simulink model "CM640A_MotAg1Meas"  (R2013b)
settings: Solver=FixedStepDiscrete  SolverMode=SingleTasking  StartTime=0.0  StopTime=1  FixedStep=0.0000625  RelTol=1e-3
undefined symbols (not defined in the file): ARCHGLBPRM_2PI_ULS_F32, COEFFTBLELMSIZE_CNT_U08, COEFFTBLSIZE_CNT_U08, CORRNTBLAGSTEPSIZE_MATRAD_F32, CORRNTBLSIDXOFFS_CNT_U16, CORRNTBLSIZE_CNT_U16, CORRNTBLSIZEMASK_CNT_U08, MOTAG1OFFS_MOTREV_U0P16, MotAg1PrtclFlt, MOTAG1PRTCLFLTFAILSTEP_CNT_U16, MOTAG1PRTCLFLTPASSSTEP_CNT_U16, MOTAGDELTAPERCORRNPT_CNT_U16, MOTAGIDXMASK_CNT_U16, MotCtrlMotAg1ErrReg, NtcSts1, sigbuilder_block, SNSRAGMASK_CNT_U32, SNSRERRMASK_CNT_U32, SNSRERRNTCMASK_CNT_U08, SNSRVLTGFLTMASK_CNT_U32, SPIPARMASK_CNT_U32
libraries: simulink x28, FloatToFixd x1, NxtrMax x1, NxtrLim x1
(part 3 of 4)

== system CM640A_MotAg1Meas/MotAg1Meas/MotAg1MeasInit1/Compute Correction Table/NVM Ok/Calculate Correction Table/Build Wave ==
  Constant : Constant  Value=CORRNTBLSIZE_CNT_U16
  CopyRight2 : Subsystem  Description=|  mask(Copyright Information){none=on}
      | Copyright info block.                                               
      |                                                                     
      | Place copyright information at the top of every subsystem in design.
      mask prompts: none "No parameters"
      mask help: Place copyright information at the top of every subsystem in design.
      mask Display:
      | NxtrConf = 'Nexteer Confidential';
      | 
      | sys = bdroot; %handle for the current model ("system")
      | first = get_param(sys,'Created');
      | first = first(end-3:end);  %year is last four digits
      | 
      | last = get_param(sys,'LastModifiedDate');
      | if isempty(last)
      |     last = datestr(now,'yyyy');
      | else
      |     last = last(end-3:end);
      | end
      | 
      | if strcmp(first,last)
      |     fprintf('%s -- Copyright %s Nexteer',NxtrConf,first)
      | else
      |     fprintf('%s -- %s%s- %s Nexteer',NxtrConf,char(169),first,last)
      | end
  Reconstructed Waveform Processing : Subsystem  TreatAsAtomicUnit=on
  wires:
  Constant/1 -> Reconstructed Waveform Processing/1(N)

== system CM640A_MotAg1Meas/MotAg1Meas/MotAg1MeasInit1/Compute Correction Table/NVM Ok/Calculate Correction Table/Change Correction Coordinate ==
  Constant1 : Constant  Value=CORRNTBLSIZE_CNT_U16
  CopyRight2 : Subsystem  Description=|  mask(Copyright Information){none=on}
      | Copyright info block.                                               
      |                                                                     
      | Place copyright information at the top of every subsystem in design.
      mask prompts: none "No parameters"
      mask help: Place copyright information at the top of every subsystem in design.
      mask Display:
      | NxtrConf = 'Nexteer Confidential';
      | 
      | sys = bdroot; %handle for the current model ("system")
      | first = get_param(sys,'Created');
      | first = first(end-3:end);  %year is last four digits
      | 
      | last = get_param(sys,'LastModifiedDate');
      | if isempty(last)
      |     last = datestr(now,'yyyy');
      | else
      |     last = last(end-3:end);
      | end
      | 
      | if strcmp(first,last)
      |     fprintf('%s -- Copyright %s Nexteer',NxtrConf,first)
      | else
      |     fprintf('%s -- %s%s- %s Nexteer',NxtrConf,char(169),first,last)
      | end
  Waveform Coordinate Change : Subsystem  TreatAsAtomicUnit=on
  wires:
  Constant1/1 -> Waveform Coordinate Change/1(N)

== system CM640A_MotAg1Meas/MotAg1Meas/MotAg1MeasInit1/Compute Correction Table/NVM Ok/Calculate Correction Table/CopyRight2 ==

== system CM640A_MotAg1Meas/MotAg1Meas/MotAg1MeasInit1/Compute Correction Table/NVM Ok/Configure Coefficients/CopyRight2 ==

== system CM640A_MotAg1Meas/MotAg1Meas/MotAg1MeasPer1/Process MotAg1 Angle/Process MotAg1Raw/MotAg Message Parity Monitoring/Atomic Subsystem2 ==
  InputBoolean : Inport  OutDataTypeStr=boolean
  If : If  IfExpression=u1 ~= 0
  Merge : Merge
  Output 0 : Subsystem  TreatAsAtomicUnit=on
  Output 1 : Subsystem  TreatAsAtomicUnit=on
  OutputNumber : Outport  OutDataTypeStr=uint8
  wires:
  InputBoolean/1 -> If/1
  If/1 -> Output 1/Action
  If/2 -> Output 0/Action
  Output 1/1(Out1) -> Merge/1
  Output 0/1(Out1) -> Merge/2
  Merge/1 -> OutputNumber/1

== system CM640A_MotAg1Meas/MotAg1Meas/MotAg1MeasPer1/Process MotAg1 Angle/Process MotAg1Raw/MotAg Message Parity Monitoring/Atomic Subsystem3 ==
  InputBoolean : Inport  OutDataTypeStr=boolean
  If : If  IfExpression=u1 ~= 0
  Merge : Merge
  Output 0 : Subsystem  TreatAsAtomicUnit=on
  Output 1 : Subsystem  TreatAsAtomicUnit=on
  OutputNumber : Outport  OutDataTypeStr=uint8
  wires:
  Merge/1 -> OutputNumber/1
  Output 0/1(Out1) -> Merge/2
  Output 1/1(Out1) -> Merge/1
  If/2 -> Output 0/Action
  If/1 -> Output 1/Action
  InputBoolean/1 -> If/1

== system CM640A_MotAg1Meas/MotAg1Meas/MotAg1MeasPer1/Process MotAg1 Angle/Process MotAg1Raw/MotAg Message Parity Monitoring/CopyRight2 ==

== system CM640A_MotAg1Meas/MotAg1Meas/MotAg1MeasPer1/Process MotAg1 Angle/Process MotAg1Raw/Raw Mecl Mot Ag Processing/CopyRight2 ==

== system CM640A_MotAg1Meas/MotAg1Meas/MotAg1MeasPer1/Process MotAg1 Angle/Process MotAg1Raw/Undervoltage Bit Monitoring/Atomic Subsystem1 ==
  InputBoolean : Inport  OutDataTypeStr=boolean
  If : If  IfExpression=u1 ~= 0
  Merge : Merge
  Output 0 : Subsystem  TreatAsAtomicUnit=on
  Output 1 : Subsystem  TreatAsAtomicUnit=on
  OutputNumber : Outport  OutDataTypeStr=uint8
  wires:
  InputBoolean/1 -> If/1
  If/1 -> Output 1/Action
  If/2 -> Output 0/Action
  Output 1/1(Out1) -> Merge/1
  Output 0/1(Out1) -> Merge/2
  Merge/1 -> OutputNumber/1

== system CM640A_MotAg1Meas/MotAg1Meas/MotAg1MeasPer1/Process MotAg1 Angle/Process MotAg1Raw/Undervoltage Bit Monitoring/CopyRight2 ==

== system CM640A_MotAg1Meas/MotAg1Meas/MotAg1MeasPer2/MotAg1 Protocol Fault Operation/Atomic Subsystem/N Step/CopyRight2 ==

== system CM640A_MotAg1Meas/MotAg1Meas/MotAg1MeasPer2/MotAg1 Protocol Fault Operation/Atomic Subsystem/P Step/CopyRight2 ==

== system CM640A_MotAg1Meas/MotAg1Meas/MotAg1MeasPer2/MotAg1 Protocol Fault Operation/Subsystem/Atomic Subsystem1/Output 0 ==
  Action Port : ActionPort  ActionType=else
  Bit 7 : Constant  Value=0  OutDataTypeStr=uint8
  Out1 : Outport  InitialOutput=0
  wires:
  Bit 7/1 -> Out1/1

== system CM640A_MotAg1Meas/MotAg1Meas/MotAg1MeasPer2/MotAg1 Protocol Fault Operation/Subsystem/Atomic Subsystem1/Output 1 ==
  Action Port : ActionPort  ActionType=then
  Bit 7 : Constant  OutDataTypeStr=uint8
  Out1 : Outport  InitialOutput=1
  wires:
  Bit 7/1 -> Out1/1

== system CM640A_MotAg1Meas/MotAg1Meas/MotAg1MeasPer2/MotAg1 Protocol Fault Operation/Subsystem/Atomic Subsystem2/Output 0 ==
  Action Port : ActionPort  ActionType=else
  Bit 7 : Constant  Value=0  OutDataTypeStr=uint8
  Out1 : Outport  InitialOutput=0
  wires:
  Bit 7/1 -> Out1/1

== system CM640A_MotAg1Meas/MotAg1Meas/MotAg1MeasPer2/MotAg1 Protocol Fault Operation/Subsystem/Atomic Subsystem2/Output 1 ==
  Action Port : ActionPort  ActionType=then
  Bit 7 : Constant  OutDataTypeStr=uint8
  Out1 : Outport  InitialOutput=1
  wires:
  Bit 7/1 -> Out1/1

== system CM640A_MotAg1Meas/MotAg1Meas/MotAg1MeasPer2/MotAg1 Protocol Fault Operation/Subsystem/Atomic Subsystem3/Output 0 ==
  Action Port : ActionPort  ActionType=else
  Bit 7 : Constant  Value=0  OutDataTypeStr=uint8
  Out1 : Outport  InitialOutput=0
  wires:
  Bit 7/1 -> Out1/1

== system CM640A_MotAg1Meas/MotAg1Meas/MotAg1MeasPer2/MotAg1 Protocol Fault Operation/Subsystem/Atomic Subsystem3/Output 1 ==
  Action Port : ActionPort  ActionType=then
  Bit 7 : Constant  OutDataTypeStr=uint8
  Out1 : Outport  InitialOutput=1
  wires:
  Bit 7/1 -> Out1/1

== system CM640A_MotAg1Meas/MotAg1Meas/MotAg1MeasPer2/Process ErrorReg and DieRevCtr/Process MotAg1RawErr/Invalid Polarity, Hold Last Value/CopyRight2 ==

== system CM640A_MotAg1Meas/MotAg1Meas/MotAg1MeasPer2/Process ErrorReg and DieRevCtr/Process MotAg1RawErr/Process MotAg1RawErr/Atomic Subsystem1 ==
  InputBoolean : Inport  OutDataTypeStr=boolean
  If : If  IfExpression=u1 ~= 0
  Merge : Merge
  Output 0 : Subsystem  TreatAsAtomicUnit=on
  Output 1 : Subsystem  TreatAsAtomicUnit=on
  OutputNumber : Outport  OutDataTypeStr=uint8
  wires:
  InputBoolean/1 -> If/1
  If/1 -> Output 1/Action
  If/2 -> Output 0/Action
  Output 1/1(Out1) -> Merge/1
  Output 0/1(Out1) -> Merge/2
  Merge/1 -> OutputNumber/1

== system CM640A_MotAg1Meas/MotAg1Meas/MotAg1MeasPer2/Process ErrorReg and DieRevCtr/Process MotAg1RawErr/Process MotAg1RawErr/Atomic Subsystem2 ==
  InputBoolean : Inport  OutDataTypeStr=boolean
  If : If  IfExpression=u1 ~= 0
  Merge : Merge
  Output 0 : Subsystem  TreatAsAtomicUnit=on
  Output 1 : Subsystem  TreatAsAtomicUnit=on
  OutputNumber : Outport  OutDataTypeStr=uint8
  wires:
  Merge/1 -> OutputNumber/1
  Output 0/1(Out1) -> Merge/2
  Output 1/1(Out1) -> Merge/1
  If/2 -> Output 0/Action
  If/1 -> Output 1/Action
  InputBoolean/1 -> If/1

== system CM640A_MotAg1Meas/MotAg1Meas/MotAg1MeasPer2/Process ErrorReg and DieRevCtr/Process MotAg1RawErr/Process MotAg1RawErr/CopyRight2 ==

== system CM640A_MotAg1Meas/MotAg1Meas/MotAg1MeasPer2/Process ErrorReg and DieRevCtr/Process MotAg1RawErr/Valid Polarity/CopyRight2 ==

== system CM640A_MotAg1Meas/MotAg1Meas/MotAg1MeasInit1/Compute Correction Table/NVM Ok/Calculate Correction Table/Build Wave/CopyRight2 ==

== system CM640A_MotAg1Meas/MotAg1Meas/MotAg1MeasInit1/Compute Correction Table/NVM Ok/Calculate Correction Table/Build Wave/Reconstructed Waveform Processing ==
  N : Inport
  Assignment : Assignment  IndexMode=Zero-based  IndexOptions=Index vector (port)  Indices=1  OutputSizes=1
  Constant : Constant  Value=COEFFTBLSIZE_CNT_U08
  Constant1 : Constant  Value=CORRNTBLAGSTEPSIZE_MATRAD_F32
  CopyRight2 : Subsystem  Description=|  mask(Copyright Information){none=on}
      | Copyright info block.                                               
      |                                                                     
      | Place copyright information at the top of every subsystem in design.
      mask prompts: none "No parameters"
      mask help: Place copyright information at the top of every subsystem in design.
      mask Display:
      | NxtrConf = 'Nexteer Confidential';
      | 
      | sys = bdroot; %handle for the current model ("system")
      | first = get_param(sys,'Created');
      | first = first(end-3:end);  %year is last four digits
      | 
      | last = get_param(sys,'LastModifiedDate');
      | if isempty(last)
      |     last = datestr(now,'yyyy');
      | else
      |     last = last(end-3:end);
      | end
      | 
      | if strcmp(first,last)
      |     fprintf('%s -- Copyright %s Nexteer',NxtrConf,first)
      | else
      |     fprintf('%s -- %s%s- %s Nexteer',NxtrConf,char(169),first,last)
      | end
  Data Store Read : DataStoreRead  DataStoreName=ReconstructedWaveform_RevM_f32
  Data Store Write : DataStoreWrite  DataStoreName=ReconstructedWaveform_RevM_f32
  Data Type Conversion : DataTypeConversion  OutDataTypeStr=single
  Data Type Conversion1 : DataTypeConversion  OutDataTypeStr=int8
  For Iterator : ForIterator  ResetStates=reset  IterationSource=external  IndexMode=Zero-based  IterationVariableDataType=int16
  Harmonic Coefficient Processing : Subsystem  TreatAsAtomicUnit=on
  Product : Product
  Subtract 1 because the first order is not included : Bias  Bias=-1
  wires:
  Constant/1 -> Data Type Conversion1/1
  N/1 -> For Iterator/1
  For Iterator/1 -> Data Type Conversion/1, Assignment/3
  Data Type Conversion/1 -> Product/1
  Constant1/1 -> Product/2
  Product/1 -> Harmonic Coefficient Processing/1(HarmAngle)
  Subtract 1 because the first order is not included/1 -> Harmonic Coefficient Processing/2(Coefficient Table Size)
  Data Type Conversion1/1 -> Subtract 1 because the first order is not included/1
  Harmonic Coefficient Processing/1(Reconstructed Waveform Element) -> Assignment/2
  Data Store Read/1 -> Assignment/1
  Assignment/1 -> Data Store Write/1

== system CM640A_MotAg1Meas/MotAg1Meas/MotAg1MeasInit1/Compute Correction Table/NVM Ok/Calculate Correction Table/Change Correction Coordinate/CopyRight2 ==

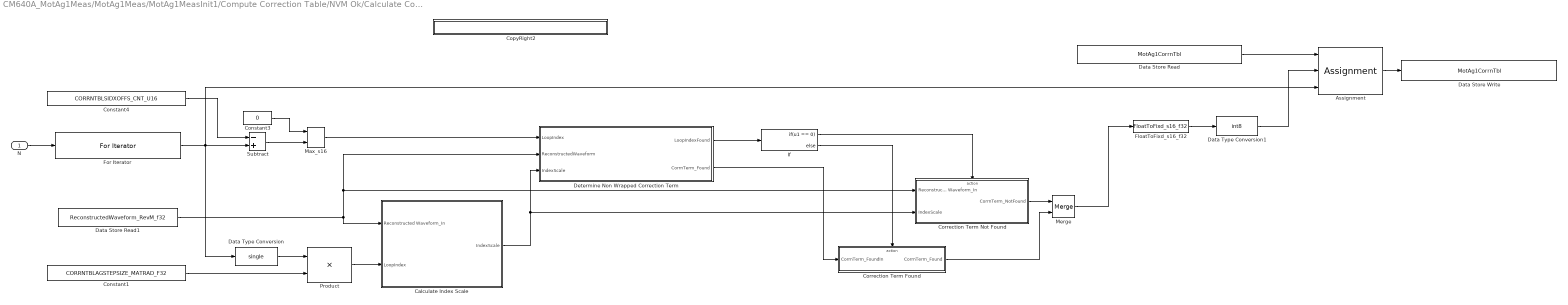
== system CM640A_MotAg1Meas/MotAg1Meas/MotAg1MeasInit1/Compute Correction Table/NVM Ok/Calculate Correction Table/Change Correction Coordinate/Waveform Coordinate Change ==
  N : Inport
  Assignment : Assignment  IndexMode=Zero-based  IndexOptions=Index vector (port)  Indices=1  OutputSizes=1
  Calculate Index Scale : Subsystem  TreatAsAtomicUnit=on
  Constant1 : Constant  Value=CORRNTBLAGSTEPSIZE_MATRAD_F32
  Constant3 : Constant  Value=0  OutDataTypeStr=int16
  Constant4 : Constant  Value=CORRNTBLSIDXOFFS_CNT_U16
  CopyRight2 : Subsystem  Description=|  mask(Copyright Information){none=on}
      | Copyright info block.                                               
      |                                                                     
      | Place copyright information at the top of every subsystem in design.
      mask prompts: none "No parameters"
      mask help: Place copyright information at the top of every subsystem in design.
      mask Display:
      | NxtrConf = 'Nexteer Confidential';
      | 
      | sys = bdroot; %handle for the current model ("system")
      | first = get_param(sys,'Created');
      | first = first(end-3:end);  %year is last four digits
      | 
      | last = get_param(sys,'LastModifiedDate');
      | if isempty(last)
      |     last = datestr(now,'yyyy');
      | else
      |     last = last(end-3:end);
      | end
      | 
      | if strcmp(first,last)
      |     fprintf('%s -- Copyright %s Nexteer',NxtrConf,first)
      | else
      |     fprintf('%s -- %s%s- %s Nexteer',NxtrConf,char(169),first,last)
      | end
  Correction Term Found : Subsystem  TreatAsAtomicUnit=on
  Correction Term Not Found : Subsystem  TreatAsAtomicUnit=on
  Data Store Read : DataStoreRead  DataStoreName=MotAg1CorrnTbl
  Data Store Read1 : DataStoreRead  DataStoreName=ReconstructedWaveform_RevM_f32
  Data Store Write : DataStoreWrite  DataStoreName=MotAg1CorrnTbl
  Data Type Conversion : DataTypeConversion  OutDataTypeStr=single
  Data Type Conversion1 : DataTypeConversion  OutDataTypeStr=int8
  Determine Non Wrapped Correction Term : Subsystem  TreatAsAtomicUnit=on
  FloatToFixd_s16_f32 : FloatToFixd/FloatToFixd_s16_f32  Param1=12
  For Iterator : ForIterator  ResetStates=reset  IterationSource=external  IndexMode=Zero-based  IterationVariableDataType=int16
  If : If  IfExpression=u1 == 0
  Max_s16 : NxtrMax/Max_s16  SFunctionSpec="int16 y1 = Max_s16( int16 u1,  int16 u2)"
      settings: AttributesFormatString=%<Name>
  Merge : Merge
  Product : Product
  Subtract : Sum  Inputs=-+  OutDataTypeStr=int16
  wires:
  Constant1/1 -> Product/2
  Data Type Conversion/1 -> Product/1
  For Iterator/1 -> Data Type Conversion/1, Assignment/3, Subtract/2
  N/1 -> For Iterator/1
  Data Store Read1/1 -> Calculate Index Scale/1(Reconstructed Waveform_In), Correction Term Not Found/1(Reconstructed Waveform_In), Determine Non Wrapped Correction Term/2(ReconstructedWaveform)
  Product/1 -> Calculate Index Scale/2(LoopIndex)
  Calculate Index Scale/1(IndexScale) -> Correction Term Not Found/2(IndexScale), Determine Non Wrapped Correction Term/3(IndexScale)
  Constant3/1 -> Max_s16/1
  Subtract/1 -> Max_s16/2
  Constant4/1 -> Subtract/1
  Max_s16/1 -> Determine Non Wrapped Correction Term/1(LoopIndex)
  Determine Non Wrapped Correction Term/1(LoopIndexFound) -> If/1
  If/1 -> Correction Term Not Found/Action
  If/2 -> Correction Term Found/Action
  Determine Non Wrapped Correction Term/2(CorrnTerm_Found) -> Correction Term Found/1(CorrnTerm_FoundIn)
  Data Store Read/1 -> Assignment/1
  Correction Term Not Found/1(CorrnTerm_NotFound) -> Merge/1
  Correction Term Found/1(CorrnTerm_Found) -> Merge/2
  Merge/1 -> FloatToFixd_s16_f32/1
  Assignment/1 -> Data Store Write/1
  FloatToFixd_s16_f32/1 -> Data Type Conversion1/1
  Data Type Conversion1/1 -> Assignment/2

== system CM640A_MotAg1Meas/MotAg1Meas/MotAg1MeasPer1/Process MotAg1 Angle/Process MotAg1Raw/MotAg Message Parity Monitoring/Atomic Subsystem2/Output 0 ==
  Action Port : ActionPort  ActionType=else
  Bit 7 : Constant  Value=0  OutDataTypeStr=uint8
  Out1 : Outport  InitialOutput=0
  wires:
  Bit 7/1 -> Out1/1

== system CM640A_MotAg1Meas/MotAg1Meas/MotAg1MeasPer1/Process MotAg1 Angle/Process MotAg1Raw/MotAg Message Parity Monitoring/Atomic Subsystem2/Output 1 ==
  Action Port : ActionPort  ActionType=then
  Bit 7 : Constant  OutDataTypeStr=uint8
  Out1 : Outport  InitialOutput=1
  wires:
  Bit 7/1 -> Out1/1

== system CM640A_MotAg1Meas/MotAg1Meas/MotAg1MeasPer1/Process MotAg1 Angle/Process MotAg1Raw/MotAg Message Parity Monitoring/Atomic Subsystem3/Output 0 ==
  Action Port : ActionPort  ActionType=else
  Bit 7 : Constant  Value=0  OutDataTypeStr=uint8
  Out1 : Outport  InitialOutput=0
  wires:
  Bit 7/1 -> Out1/1

== system CM640A_MotAg1Meas/MotAg1Meas/MotAg1MeasPer1/Process MotAg1 Angle/Process MotAg1Raw/MotAg Message Parity Monitoring/Atomic Subsystem3/Output 1 ==
  Action Port : ActionPort  ActionType=then
  Bit 7 : Constant  OutDataTypeStr=uint8
  Out1 : Outport  InitialOutput=1
  wires:
  Bit 7/1 -> Out1/1

== system CM640A_MotAg1Meas/MotAg1Meas/MotAg1MeasPer1/Process MotAg1 Angle/Process MotAg1Raw/Undervoltage Bit Monitoring/Atomic Subsystem1/Output 0 ==
  Action Port : ActionPort  ActionType=else
  Bit 7 : Constant  Value=0  OutDataTypeStr=uint8
  Out1 : Outport  InitialOutput=0
  wires:
  Bit 7/1 -> Out1/1

== system CM640A_MotAg1Meas/MotAg1Meas/MotAg1MeasPer1/Process MotAg1 Angle/Process MotAg1Raw/Undervoltage Bit Monitoring/Atomic Subsystem1/Output 1 ==
  Action Port : ActionPort  ActionType=then
  Bit 7 : Constant  OutDataTypeStr=uint8
  Out1 : Outport  InitialOutput=1
  wires:
  Bit 7/1 -> Out1/1

== system CM640A_MotAg1Meas/MotAg1Meas/MotAg1MeasPer2/Process ErrorReg and DieRevCtr/Process MotAg1RawErr/Process MotAg1RawErr/Atomic Subsystem1/Output 0 ==
  Action Port : ActionPort  ActionType=else
  Bit 7 : Constant  Value=0  OutDataTypeStr=uint8
  Out1 : Outport  InitialOutput=0
  wires:
  Bit 7/1 -> Out1/1

== system CM640A_MotAg1Meas/MotAg1Meas/MotAg1MeasPer2/Process ErrorReg and DieRevCtr/Process MotAg1RawErr/Process MotAg1RawErr/Atomic Subsystem1/Output 1 ==
  Action Port : ActionPort  ActionType=then
  Bit 7 : Constant  OutDataTypeStr=uint8
  Out1 : Outport  InitialOutput=1
  wires:
  Bit 7/1 -> Out1/1

== system CM640A_MotAg1Meas/MotAg1Meas/MotAg1MeasPer2/Process ErrorReg and DieRevCtr/Process MotAg1RawErr/Process MotAg1RawErr/Atomic Subsystem2/Output 0 ==
  Action Port : ActionPort  ActionType=else
  Bit 7 : Constant  Value=0  OutDataTypeStr=uint8
  Out1 : Outport  InitialOutput=0
  wires:
  Bit 7/1 -> Out1/1

== system CM640A_MotAg1Meas/MotAg1Meas/MotAg1MeasPer2/Process ErrorReg and DieRevCtr/Process MotAg1RawErr/Process MotAg1RawErr/Atomic Subsystem2/Output 1 ==
  Action Port : ActionPort  ActionType=then
  Bit 7 : Constant  OutDataTypeStr=uint8
  Out1 : Outport  InitialOutput=1
  wires:
  Bit 7/1 -> Out1/1

== system CM640A_MotAg1Meas/MotAg1Meas/MotAg1MeasInit1/Compute Correction Table/NVM Ok/Calculate Correction Table/Build Wave/Reconstructed Waveform Processing/CopyRight2 ==

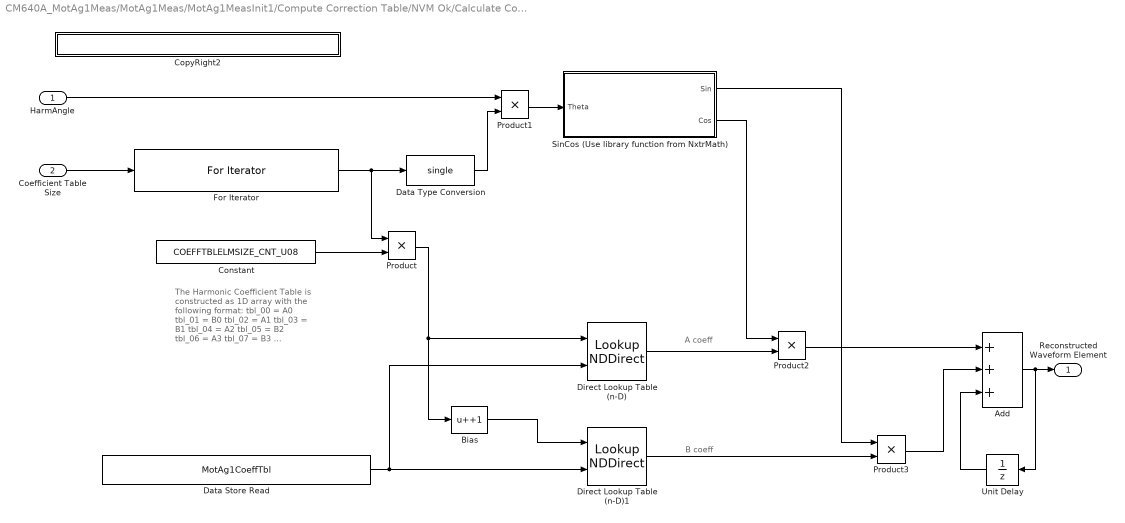
== system CM640A_MotAg1Meas/MotAg1Meas/MotAg1MeasInit1/Compute Correction Table/NVM Ok/Calculate Correction Table/Build Wave/Reconstructed Waveform Processing/Harmonic Coefficient Processing ==
  note: B coeff
  note: A coeff
  note: The Harmonic Coefficient Table
      | is constructed as 1D array with
      | the following format:
      |
      | tbl_00 = A0
      | tbl_01 = B0
      | tbl_02 = A1
      | tbl_03 = B1
      | tbl_04 = A2
      | tbl_05 = B2
      | tbl_06 = A3
      | tbl_07 = B3
      | ...
  HarmAngle : Inport
  Coefficient Table Size : Inport  Port=2
  Add : Sum  Inputs=+++
  Bias : Bias  Bias=+1
  Constant : Constant  Value=COEFFTBLELMSIZE_CNT_U08
  CopyRight2 : Subsystem  Description=|  mask(Copyright Information){none=on}
      | Copyright info block.                                               
      |                                                                     
      | Place copyright information at the top of every subsystem in design.
      mask prompts: none "No parameters"
      mask help: Place copyright information at the top of every subsystem in design.
      mask Display:
      | NxtrConf = 'Nexteer Confidential';
      | 
      | sys = bdroot; %handle for the current model ("system")
      | first = get_param(sys,'Created');
      | first = first(end-3:end);  %year is last four digits
      | 
      | last = get_param(sys,'LastModifiedDate');
      | if isempty(last)
      |     last = datestr(now,'yyyy');
      | else
      |     last = last(end-3:end);
      | end
      | 
      | if strcmp(first,last)
      |     fprintf('%s -- Copyright %s Nexteer',NxtrConf,first)
      | else
      |     fprintf('%s -- %s%s- %s Nexteer',NxtrConf,char(169),first,last)
      | end
  Data Store Read : DataStoreRead  DataStoreName=MotAg1CoeffTbl
  Data Type Conversion : DataTypeConversion  OutDataTypeStr=single
  Direct Lookup Table (n-D) : LookupNDDirect  NumberOfTableDimensions=1  TableIsInput=on
  Direct Lookup Table (n-D)1 : LookupNDDirect  NumberOfTableDimensions=1  TableIsInput=on
  For Iterator : ForIterator  ResetStates=reset  IterationSource=external  IterationVariableDataType=int8
  Product{,1..3} (4 alike) : Product
  SinCos (Use library function from NxtrMath) : Subsystem  TreatAsAtomicUnit=on
  Unit Delay : UnitDelay  SampleTime=-1
  Reconstructed Waveform Element : Outport
  wires:
  Coefficient Table Size/1 -> For Iterator/1
  Data Store Read/1 -> Direct Lookup Table (n-D)/2, Direct Lookup Table (n-D)1/2
  Constant/1 -> Product/2
  For Iterator/1 -> Data Type Conversion/1, Product/1
  HarmAngle/1 -> Product1/1
  Data Type Conversion/1 -> Product1/2
  Product1/1 -> SinCos (Use library function from NxtrMath)/1(Theta)
  Product/1 -> Bias/1, Direct Lookup Table (n-D)/1
  Bias/1 -> Direct Lookup Table (n-D)1/1
  SinCos (Use library function from NxtrMath)/2(Cos) -> Product2/1
  Direct Lookup Table (n-D)/1 -> Product2/2
  Direct Lookup Table (n-D)1/1 -> Product3/2
  SinCos (Use library function from NxtrMath)/1(Sin) -> Product3/1
  Product2/1 -> Add/1
  Product3/1 -> Add/2
  Unit Delay/1 -> Add/3
  Add/1 -> Unit Delay/1, Reconstructed Waveform Element/1

== system CM640A_MotAg1Meas/MotAg1Meas/MotAg1MeasInit1/Compute Correction Table/NVM Ok/Calculate Correction Table/Change Correction Coordinate/Waveform Coordinate Change/Calculate Index Scale ==
  Reconstructed Waveform_In : Inport
  LoopIndex : Inport  Port=2
  CopyRight2 : Subsystem  Description=|  mask(Copyright Information){none=on}
      | Copyright info block.                                               
      |                                                                     
      | Place copyright information at the top of every subsystem in design.
      mask prompts: none "No parameters"
      mask help: Place copyright information at the top of every subsystem in design.
      mask Display:
      | NxtrConf = 'Nexteer Confidential';
      | 
      | sys = bdroot; %handle for the current model ("system")
      | first = get_param(sys,'Created');
      | first = first(end-3:end);  %year is last four digits
      | 
      | last = get_param(sys,'LastModifiedDate');
      | if isempty(last)
      |     last = datestr(now,'yyyy');
      | else
      |     last = last(end-3:end);
      | end
      | 
      | if strcmp(first,last)
      |     fprintf('%s -- Copyright %s Nexteer',NxtrConf,first)
      | else
      |     fprintf('%s -- %s%s- %s Nexteer',NxtrConf,char(169),first,last)
      | end
  Direct Lookup Table (n-D) : LookupNDDirect  NumberOfTableDimensions=1  TableIsInput=on
  First Entry Index : Constant  Value=0
  First Entry Index1 : Constant  Value=ARCHGLBPRM_2PI_ULS_F32
  Truth Table : Truth Table  TreatAsAtomicUnit=on
  IndexScale : Outport
  wires:
  Reconstructed Waveform_In/1 -> Direct Lookup Table (n-D)/2
  First Entry Index/1 -> Direct Lookup Table (n-D)/1
  Direct Lookup Table (n-D)/1 -> Truth Table/1(ReconWfrm_0)
  LoopIndex/1 -> Truth Table/2(LoopIndex)
  First Entry Index1/1 -> Truth Table/3(ARCHGLBPRM_2PI_ULS_F32)
  Truth Table/1(IndexScale) -> IndexScale/1

== system CM640A_MotAg1Meas/MotAg1Meas/MotAg1MeasInit1/Compute Correction Table/NVM Ok/Calculate Correction Table/Change Correction Coordinate/Waveform Coordinate Change/CopyRight2 ==

== system CM640A_MotAg1Meas/MotAg1Meas/MotAg1MeasInit1/Compute Correction Table/NVM Ok/Calculate Correction Table/Change Correction Coordinate/Waveform Coordinate Change/Correction Term Found ==
  CorrnTerm_FoundIn : Inport
  Action Port : ActionPort  ActionType=else
  CopyRight2 : Subsystem  Description=|  mask(Copyright Information){none=on}
      | Copyright info block.                                               
      |                                                                     
      | Place copyright information at the top of every subsystem in design.
      mask prompts: none "No parameters"
      mask help: Place copyright information at the top of every subsystem in design.
      mask Display:
      | NxtrConf = 'Nexteer Confidential';
      | 
      | sys = bdroot; %handle for the current model ("system")
      | first = get_param(sys,'Created');
      | first = first(end-3:end);  %year is last four digits
      | 
      | last = get_param(sys,'LastModifiedDate');
      | if isempty(last)
      |     last = datestr(now,'yyyy');
      | else
      |     last = last(end-3:end);
      | end
      | 
      | if strcmp(first,last)
      |     fprintf('%s -- Copyright %s Nexteer',NxtrConf,first)
      | else
      |     fprintf('%s -- %s%s- %s Nexteer',NxtrConf,char(169),first,last)
      | end
  CorrnTerm_Found : Outport
  wires:
  CorrnTerm_FoundIn/1 -> CorrnTerm_Found/1

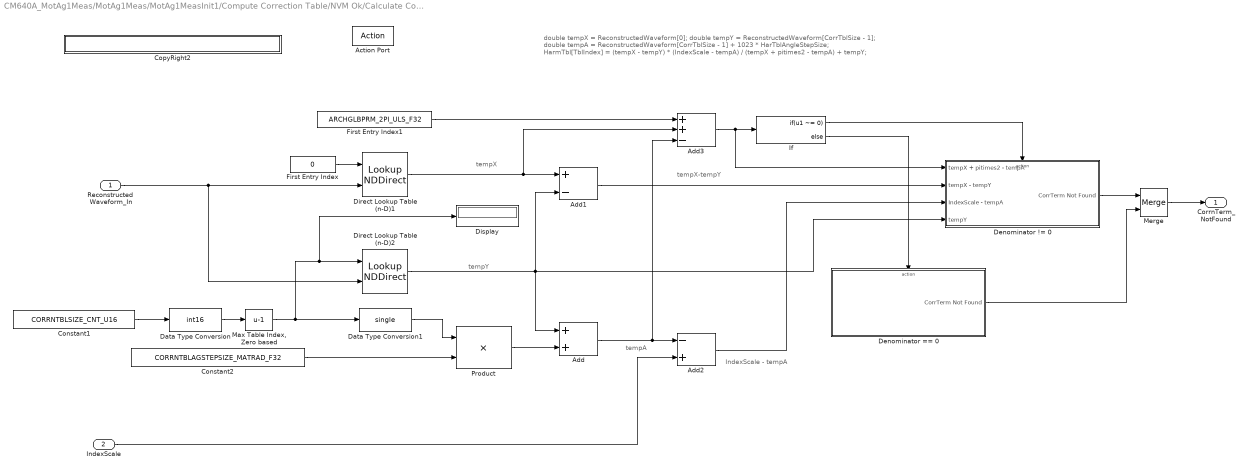
== system CM640A_MotAg1Meas/MotAg1Meas/MotAg1MeasInit1/Compute Correction Table/NVM Ok/Calculate Correction Table/Change Correction Coordinate/Waveform Coordinate Change/Correction Term Not Found ==
  note: double tempX = ReconstructedWaveform[0];
      | double tempY = ReconstructedWaveform[CorrTblSize - 1];
      | double tempA = ReconstructedWaveform[CorrTblSize - 1] + 1023 * HarTblAngleStepSize;
      |
      | HarmTbl[TblIndex] = (tempX - tempY) * (IndexScale - tempA) / (tempX + pitimes2 - tempA) + tempY;
  note: tempX-tempY
  note: IndexScale - tempA
  note: tempA
  note: tempX
  note: tempY
  Reconstructed Waveform_In : Inport  OutDataTypeStr=single
  IndexScale : Inport  Port=2
  Action Port : ActionPort  ActionType=then
  Add : Sum
  Add1 : Sum  Inputs=+-
  Add2 : Sum  Inputs=-+
  Add3 : Sum  Inputs=++-
  Constant1 : Constant  Value=CORRNTBLSIZE_CNT_U16
  Constant2 : Constant  Value=CORRNTBLAGSTEPSIZE_MATRAD_F32
  CopyRight2 : Subsystem  Description=|  mask(Copyright Information){none=on}
      | Copyright info block.                                               
      |                                                                     
      | Place copyright information at the top of every subsystem in design.
      mask prompts: none "No parameters"
      mask help: Place copyright information at the top of every subsystem in design.
      mask Display:
      | NxtrConf = 'Nexteer Confidential';
      | 
      | sys = bdroot; %handle for the current model ("system")
      | first = get_param(sys,'Created');
      | first = first(end-3:end);  %year is last four digits
      | 
      | last = get_param(sys,'LastModifiedDate');
      | if isempty(last)
      |     last = datestr(now,'yyyy');
      | else
      |     last = last(end-3:end);
      | end
      | 
      | if strcmp(first,last)
      |     fprintf('%s -- Copyright %s Nexteer',NxtrConf,first)
      | else
      |     fprintf('%s -- %s%s- %s Nexteer',NxtrConf,char(169),first,last)
      | end
  Data Type Conversion : DataTypeConversion  OutDataTypeStr=int16
  Data Type Conversion1 : DataTypeConversion  OutDataTypeStr=single
  Denominator != 0 : Subsystem  TreatAsAtomicUnit=on
  Denominator == 0 : Subsystem  TreatAsAtomicUnit=on
  Direct Lookup Table (n-D)1 : LookupNDDirect  NumberOfTableDimensions=1  TableIsInput=on
  Direct Lookup Table (n-D)2 : LookupNDDirect  NumberOfTableDimensions=1  TableIsInput=on
  Display : Display
  First Entry Index : Constant  Value=0
  First Entry Index1 : Constant  Value=ARCHGLBPRM_2PI_ULS_F32
  If : If  IfExpression=u1 ~= 0
  "Max Table Index, Zero based" : Bias  Bias=-1
  Merge : Merge
  Product : Product
  CorrnTerm_NotFound : Outport
  wires:
  Reconstructed Waveform_In/1 -> Direct Lookup Table (n-D)2/2, Direct Lookup Table (n-D)1/2
  First Entry Index/1 -> Direct Lookup Table (n-D)1/1
  Constant2/1 -> Product/2
  Constant1/1 -> Data Type Conversion/1
  "Max Table Index, Zero based"/1 -> Data Type Conversion1/1, Display/1, Direct Lookup Table (n-D)2/1
  Data Type Conversion/1 -> "Max Table Index, Zero based"/1
  Data Type Conversion1/1 -> Product/1
  Product/1 -> Add/2
  Direct Lookup Table (n-D)1/1 -> Add3/2, Add1/1
  Add/1 -> Add3/3, Add2/1
  IndexScale/1 -> Add2/2
  First Entry Index1/1 -> Add3/1
  Direct Lookup Table (n-D)2/1 -> Add/1, Denominator != 0/4(tempY), Add1/2
  Add2/1 -> Denominator != 0/3(IndexScale - tempA)
  Add1/1 -> Denominator != 0/2(tempX - tempY)
  Add3/1 -> If/1, Denominator != 0/1(tempX + pitimes2 - tempA)
  If/1 -> Denominator != 0/Action
  If/2 -> Denominator == 0/Action
  Denominator == 0/1(CorrTerm Not Found) -> Merge/2
  Denominator != 0/1(CorrTerm Not Found) -> Merge/1
  Merge/1 -> CorrnTerm_NotFound/1

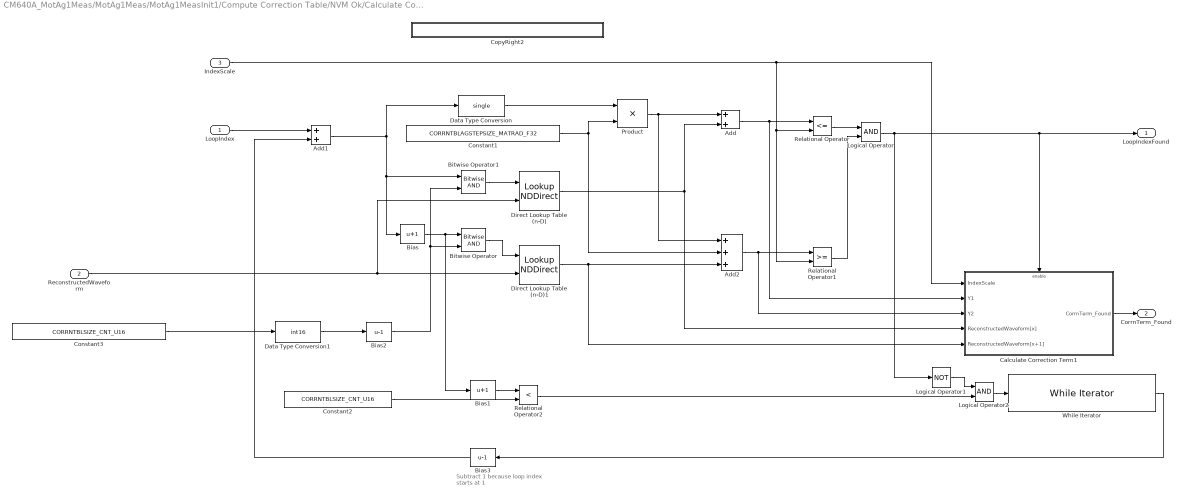
== system CM640A_MotAg1Meas/MotAg1Meas/MotAg1MeasInit1/Compute Correction Table/NVM Ok/Calculate Correction Table/Change Correction Coordinate/Waveform Coordinate Change/Determine Non Wrapped Correction Term ==
  note: Subtract 1 because
      | loop index starts at 1
  LoopIndex : Inport
  ReconstructedWaveform : Inport  Port=2
  IndexScale : Inport  Port=3
  Add : Sum
  Add1 : Sum
  Add2 : Sum  Inputs=+++
  Bias : Bias  Bias=1
  Bias1 : Bias  Bias=1
  Bias2 : Bias  Bias=-1
  Bias3 : Bias  Bias=-1
  Bitwise Operator : simulink/Logic and Bit Operations/Bitwise Operator  logicop=AND  UseBitMask=off  NumInputPorts=2  BitMask=CORRNTBLSIZE_CNT_U16-1  BitMaskRealWorld=Stored Integer
  Bitwise Operator1 : simulink/Logic and Bit Operations/Bitwise Operator  logicop=AND  UseBitMask=off  NumInputPorts=2  BitMask=CORRNTBLSIZE_CNT_U16-1  BitMaskRealWorld=Stored Integer
  Calculate Correction Term1 : Subsystem  TreatAsAtomicUnit=on
  Constant1 : Constant  Value=CORRNTBLAGSTEPSIZE_MATRAD_F32
  Constant2 : Constant  Value=CORRNTBLSIZE_CNT_U16
  Constant3 : Constant  Value=CORRNTBLSIZE_CNT_U16
  CopyRight2 : Subsystem  Description=|  mask(Copyright Information){none=on}
      | Copyright info block.                                               
      |                                                                     
      | Place copyright information at the top of every subsystem in design.
      mask prompts: none "No parameters"
      mask help: Place copyright information at the top of every subsystem in design.
      mask Display:
      | NxtrConf = 'Nexteer Confidential';
      | 
      | sys = bdroot; %handle for the current model ("system")
      | first = get_param(sys,'Created');
      | first = first(end-3:end);  %year is last four digits
      | 
      | last = get_param(sys,'LastModifiedDate');
      | if isempty(last)
      |     last = datestr(now,'yyyy');
      | else
      |     last = last(end-3:end);
      | end
      | 
      | if strcmp(first,last)
      |     fprintf('%s -- Copyright %s Nexteer',NxtrConf,first)
      | else
      |     fprintf('%s -- %s%s- %s Nexteer',NxtrConf,char(169),first,last)
      | end
  Data Type Conversion : DataTypeConversion  OutDataTypeStr=single
  Data Type Conversion1 : DataTypeConversion  OutDataTypeStr=int16
  Direct Lookup Table (n-D) : LookupNDDirect  NumberOfTableDimensions=1  TableIsInput=on
  Direct Lookup Table (n-D)1 : LookupNDDirect  NumberOfTableDimensions=1  TableIsInput=on
  Logical Operator : Logic  AllPortsSameDT=off  OutDataTypeStr=boolean
  Logical Operator1 : Logic  Operator=NOT  AllPortsSameDT=off  OutDataTypeStr=boolean
  Logical Operator2 : Logic  AllPortsSameDT=off  OutDataTypeStr=boolean
  Product : Product
  Relational Operator : RelationalOperator  Operator=<=  OutDataTypeStr=boolean
  Relational Operator1 : RelationalOperator  OutDataTypeStr=boolean
  Relational Operator2 : RelationalOperator  Operator=<  OutDataTypeStr=boolean
  While Iterator : WhileIterator  MaxIters=128  WhileBlockType=do-while  ShowIterationPort=on  OutputDataType=int16
      settings: AttributesFormatString=|
      | Max Iterations:
      | %<MaxIters>
      | (CORRNTBLSIZE_CNT_U16)
  LoopIndexFound : Outport
  CorrnTerm_Found : Outport  Port=2
  wires:
  ReconstructedWaveform/1 -> Direct Lookup Table (n-D)/2, Direct Lookup Table (n-D)1/2
  Add1/1 -> Data Type Conversion/1, Bias/1, Bitwise Operator1/1
  Bias/1 -> Bias1/1, Bitwise Operator/1
  Data Type Conversion/1 -> Product/1
  Product/1 -> Add2/1, Add/1
  Direct Lookup Table (n-D)/1 -> Calculate Correction Term1/4(ReconstructedWaveform[x]), Add/2
  LoopIndex/1 -> Add1/1
  Constant1/1 -> Add2/2, Product/2
  Direct Lookup Table (n-D)1/1 -> Calculate Correction Term1/5(ReconstructedWaveform[x+1]), Add2/3
  Add/1 -> Calculate Correction Term1/2(Y1), Relational Operator/1
  IndexScale/1 -> Calculate Correction Term1/1(IndexScale), Relational Operator1/2, Relational Operator/2
  Add2/1 -> Calculate Correction Term1/3(Y2), Relational Operator1/1
  Relational Operator/1 -> Logical Operator/1
  Relational Operator1/1 -> Logical Operator/2
  Logical Operator/1 -> LoopIndexFound/1, Calculate Correction Term1/Enable, Logical Operator1/1
  Bitwise Operator/1 -> Direct Lookup Table (n-D)1/1
  Bitwise Operator1/1 -> Direct Lookup Table (n-D)/1
  Calculate Correction Term1/1(CorrnTerm_Found) -> CorrnTerm_Found/1
  Logical Operator1/1 -> Logical Operator2/1
  Relational Operator2/1 -> Logical Operator2/2
  Logical Operator2/1 -> While Iterator/1
  Constant2/1 -> Relational Operator2/2
  Bias1/1 -> Relational Operator2/1
  While Iterator/1 -> Bias3/1
  Bias3/1 -> Add1/2
  Constant3/1 -> Data Type Conversion1/1
  Data Type Conversion1/1 -> Bias2/1
  Bias2/1 -> Bitwise Operator1/2, Bitwise Operator/2

== system CM640A_MotAg1Meas/MotAg1Meas/MotAg1MeasInit1/Compute Correction Table/NVM Ok/Calculate Correction Table/Build Wave/Reconstructed Waveform Processing/Harmonic Coefficient Processing/CopyRight2 ==

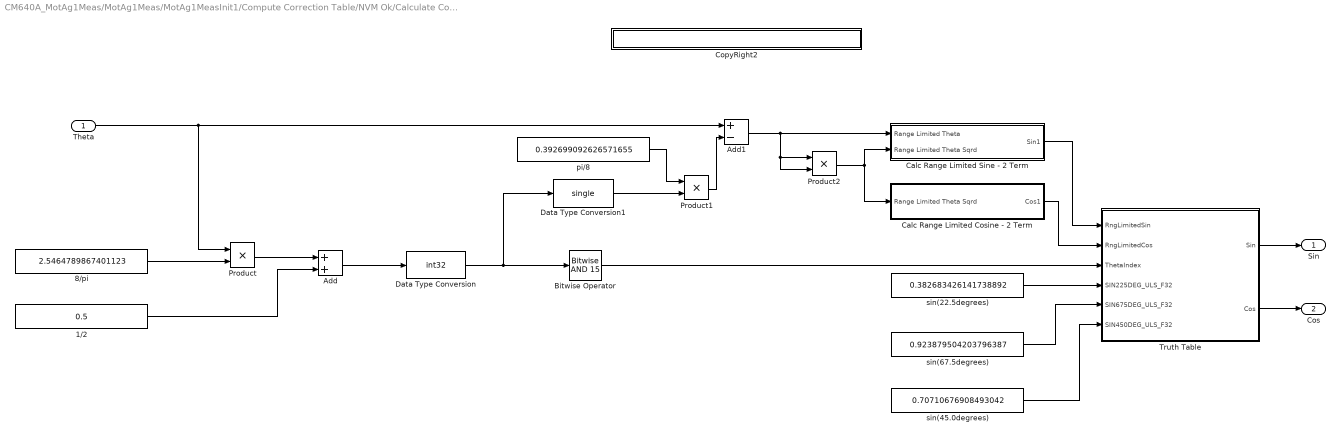
== system CM640A_MotAg1Meas/MotAg1Meas/MotAg1MeasInit1/Compute Correction Table/NVM Ok/Calculate Correction Table/Build Wave/Reconstructed Waveform Processing/Harmonic Coefficient Processing/SinCos (Use library function from NxtrMath) ==
  Theta : Inport
  1/2 : Constant  Value=0.5  OutDataTypeStr=single
  8/pi : Constant  Value=2.5464789867401123  OutDataTypeStr=single
  Add : Sum
  Add1 : Sum  Inputs=+-
  Bitwise Operator : simulink/Logic and Bit Operations/Bitwise Operator  logicop=AND  UseBitMask=on  BitMask=15  BitMaskRealWorld=Stored Integer
      settings: AttributesFormatString=|
      | BitMask:
      | %<BitMask>
  Calc Range Limited Cosine - 2 Term : Subsystem  TreatAsAtomicUnit=on
  Calc Range Limited Sine - 2 Term : Subsystem  TreatAsAtomicUnit=on
  CopyRight2 : Subsystem  Description=|  mask(Copyright Information){none=on}
      | Copyright info block.                                               
      |                                                                     
      | Place copyright information at the top of every subsystem in design.
      mask prompts: none "No parameters"
      mask help: Place copyright information at the top of every subsystem in design.
      mask Display:
      | NxtrConf = 'Nexteer Confidential';
      | 
      | sys = bdroot; %handle for the current model ("system")
      | first = get_param(sys,'Created');
      | first = first(end-3:end);  %year is last four digits
      | 
      | last = get_param(sys,'LastModifiedDate');
      | if isempty(last)
      |     last = datestr(now,'yyyy');
      | else
      |     last = last(end-3:end);
      | end
      | 
      | if strcmp(first,last)
      |     fprintf('%s -- Copyright %s Nexteer',NxtrConf,first)
      | else
      |     fprintf('%s -- %s%s- %s Nexteer',NxtrConf,char(169),first,last)
      | end
  Data Type Conversion : DataTypeConversion  OutDataTypeStr=int32
      settings: AttributesFormatString=Round Method: %<RndMeth>
  Data Type Conversion1 : DataTypeConversion  OutDataTypeStr=single
      settings: AttributesFormatString=Round Method: %<RndMeth>
  Product : Product
  Product1 : Product
  Product2 : Product
  Truth Table : Truth Table  TreatAsAtomicUnit=on
  pi/8 : Constant  Value=0.392699092626571655  OutDataTypeStr=single
  sin(22.5degrees) : Constant  Value=0.382683426141738892  OutDataTypeStr=single
  sin(45.0degrees) : Constant  Value=0.70710676908493042  OutDataTypeStr=single
  sin(67.5degrees) : Constant  Value=0.923879504203796387  OutDataTypeStr=single
  Sin : Outport
  Cos : Outport  Port=2
  wires:
  Theta/1 -> Product/1, Add1/1
  8/pi/1 -> Product/2
  Product/1 -> Add/1
  1/2/1 -> Add/2
  Add/1 -> Data Type Conversion/1
  Data Type Conversion/1 -> Data Type Conversion1/1, Bitwise Operator/1
  pi/8/1 -> Product1/1
  Data Type Conversion1/1 -> Product1/2
  Add1/1 -> Product2/2, Product2/1, Calc Range Limited Sine - 2 Term/1(Range Limited Theta)
  Product1/1 -> Add1/2
  Truth Table/1(Sin) -> Sin/1
  Bitwise Operator/1 -> Truth Table/3(ThetaIndex)
  sin(22.5degrees)/1 -> Truth Table/4(SIN225DEG_ULS_F32)
  sin(67.5degrees)/1 -> Truth Table/5(SIN675DEG_ULS_F32)
  sin(45.0degrees)/1 -> Truth Table/6(SIN450DEG_ULS_F32)
  Product2/1 -> Calc Range Limited Sine - 2 Term/2(Range Limited Theta Sqrd), Calc Range Limited Cosine - 2 Term/1(Range Limited Theta Sqrd)
  Truth Table/2(Cos) -> Cos/1
  Calc Range Limited Sine - 2 Term/1(Sin1) -> Truth Table/1(RngLimitedSin)
  Calc Range Limited Cosine - 2 Term/1(Cos1) -> Truth Table/2(RngLimitedCos)

== system CM640A_MotAg1Meas/MotAg1Meas/MotAg1MeasInit1/Compute Correction Table/NVM Ok/Calculate Correction Table/Change Correction Coordinate/Waveform Coordinate Change/Calculate Index Scale/CopyRight2 ==

== system CM640A_MotAg1Meas/MotAg1Meas/MotAg1MeasInit1/Compute Correction Table/NVM Ok/Calculate Correction Table/Change Correction Coordinate/Waveform Coordinate Change/Correction Term Found/CopyRight2 ==

== system CM640A_MotAg1Meas/MotAg1Meas/MotAg1MeasInit1/Compute Correction Table/NVM Ok/Calculate Correction Table/Change Correction Coordinate/Waveform Coordinate Change/Correction Term Not Found/CopyRight2 ==

== system CM640A_MotAg1Meas/MotAg1Meas/MotAg1MeasInit1/Compute Correction Table/NVM Ok/Calculate Correction Table/Change Correction Coordinate/Waveform Coordinate Change/Correction Term Not Found/Denominator != 0 ==
  note: (tempX - tempY) * (IndexScale - tempA) / (tempX + pitimes2 - tempA)
  note: tempY
  tempX + pitimes2 - tempA : Inport
  tempX - tempY : Inport  Port=2
  IndexScale - tempA : Inport  Port=3
  tempY : Inport  Port=4
  Action Port : ActionPort  ActionType=then
  Add4 : Sum
  CopyRight2 : Subsystem  Description=|  mask(Copyright Information){none=on}
      | Copyright info block.                                               
      |                                                                     
      | Place copyright information at the top of every subsystem in design.
      mask prompts: none "No parameters"
      mask help: Place copyright information at the top of every subsystem in design.
      mask Display:
      | NxtrConf = 'Nexteer Confidential';
      | 
      | sys = bdroot; %handle for the current model ("system")
      | first = get_param(sys,'Created');
      | first = first(end-3:end);  %year is last four digits
      | 
      | last = get_param(sys,'LastModifiedDate');
      | if isempty(last)
      |     last = datestr(now,'yyyy');
      | else
      |     last = last(end-3:end);
      | end
      | 
      | if strcmp(first,last)
      |     fprintf('%s -- Copyright %s Nexteer',NxtrConf,first)
      | else
      |     fprintf('%s -- %s%s- %s Nexteer',NxtrConf,char(169),first,last)
      | end
  "Max Table Index, Zero based1" : Bias
  Product2 : Product  Inputs=/**
  CorrTerm Not Found : Outport
  wires:
  Product2/1 -> Add4/1
  Add4/1 -> "Max Table Index, Zero based1"/1
  "Max Table Index, Zero based1"/1 -> CorrTerm Not Found/1
  tempX + pitimes2 - tempA/1 -> Product2/1
  tempX - tempY/1 -> Product2/2
  IndexScale - tempA/1 -> Product2/3
  tempY/1 -> Add4/2

== system CM640A_MotAg1Meas/MotAg1Meas/MotAg1MeasInit1/Compute Correction Table/NVM Ok/Calculate Correction Table/Change Correction Coordinate/Waveform Coordinate Change/Correction Term Not Found/Denominator == 0 ==
  Action Port : ActionPort  ActionType=else
  Constant : Constant  Value=0  OutDataTypeStr=single
  CopyRight2 : Subsystem  Description=|  mask(Copyright Information){none=on}
      | Copyright info block.                                               
      |                                                                     
      | Place copyright information at the top of every subsystem in design.
      mask prompts: none "No parameters"
      mask help: Place copyright information at the top of every subsystem in design.
      mask Display:
      | NxtrConf = 'Nexteer Confidential';
      | 
      | sys = bdroot; %handle for the current model ("system")
      | first = get_param(sys,'Created');
      | first = first(end-3:end);  %year is last four digits
      | 
      | last = get_param(sys,'LastModifiedDate');
      | if isempty(last)
      |     last = datestr(now,'yyyy');
      | else
      |     last = last(end-3:end);
      | end
      | 
      | if strcmp(first,last)
      |     fprintf('%s -- Copyright %s Nexteer',NxtrConf,first)
      | else
      |     fprintf('%s -- %s%s- %s Nexteer',NxtrConf,char(169),first,last)
      | end
  CorrTerm Not Found : Outport
  wires:
  Constant/1 -> CorrTerm Not Found/1

== system CM640A_MotAg1Meas/MotAg1Meas/MotAg1MeasInit1/Compute Correction Table/NVM Ok/Calculate Correction Table/Change Correction Coordinate/Waveform Coordinate Change/Determine Non Wrapped Correction Term/Calculate Correction Term1 ==
  IndexScale : Inport
  Y1 : Inport  Port=2
  Y2 : Inport  Port=3
  ReconstructedWaveform[x] : Inport  Port=4
  ReconstructedWaveform[x+1] : Inport  Port=5
  Enable : EnablePort
  Calculate Correction Term : Subsystem  TreatAsAtomicUnit=on
  CopyRight2 : Subsystem  Description=|  mask(Copyright Information){none=on}
      | Copyright info block.                                               
      |                                                                     
      | Place copyright information at the top of every subsystem in design.
      mask prompts: none "No parameters"
      mask help: Place copyright information at the top of every subsystem in design.
      mask Display:
      | NxtrConf = 'Nexteer Confidential';
      | 
      | sys = bdroot; %handle for the current model ("system")
      | first = get_param(sys,'Created');
      | first = first(end-3:end);  %year is last four digits
      | 
      | last = get_param(sys,'LastModifiedDate');
      | if isempty(last)
      |     last = datestr(now,'yyyy');
      | else
      |     last = last(end-3:end);
      | end
      | 
      | if strcmp(first,last)
      |     fprintf('%s -- Copyright %s Nexteer',NxtrConf,first)
      | else
      |     fprintf('%s -- %s%s- %s Nexteer',NxtrConf,char(169),first,last)
      | end
  Denominator == 0 : Subsystem  TreatAsAtomicUnit=on
  If : If  NumInputs=2  IfExpression=u1 == u2
  Merge : Merge
  CorrnTerm_Found : Outport
  wires:
  If/2 -> Calculate Correction Term/Action
  If/1 -> Denominator == 0/Action
  ReconstructedWaveform[x]/1 -> Calculate Correction Term/4(ReconstructedWaveform[x])
  ReconstructedWaveform[x+1]/1 -> Calculate Correction Term/5(ReconstructedWaveform[x+1])
  Y1/1 -> Calculate Correction Term/1(Y1), If/1
  Y2/1 -> If/2, Calculate Correction Term/2(Y2)
  IndexScale/1 -> Calculate Correction Term/3(IndexScale)
  Denominator == 0/1(CorrTerm Found) -> Merge/1
  Calculate Correction Term/1(CorrnTerm_Found) -> Merge/2
  Merge/1 -> CorrnTerm_Found/1

== system CM640A_MotAg1Meas/MotAg1Meas/MotAg1MeasInit1/Compute Correction Table/NVM Ok/Calculate Correction Table/Change Correction Coordinate/Waveform Coordinate Change/Determine Non Wrapped Correction Term/CopyRight2 ==

== system CM640A_MotAg1Meas/MotAg1Meas/MotAg1MeasInit1/Compute Correction Table/NVM Ok/Calculate Correction Table/Build Wave/Reconstructed Waveform Processing/Harmonic Coefficient Processing/SinCos (Use library function from NxtrMath)/Calc Range Limited Cosine - 2 Term ==
  note: This block calculates the taylor series of cos to 2 terms
      |
      | Cos(x) = 1 - X^2/2!
      | Cos(x) = 1 - X^2/2
  note: X^2
  note: 1/2
  note: X^2 * (1/2)
  note: 1 - X^2 * (1/2)
  Range Limited Theta Sqrd : Inport
  CopyRight2 : Subsystem  Description=|  mask(Copyright Information){none=on}
      | Copyright info block.                                               
      |                                                                     
      | Place copyright information at the top of every subsystem in design.
      mask prompts: none "No parameters"
      mask help: Place copyright information at the top of every subsystem in design.
      mask Display:
      | NxtrConf = 'Nexteer Confidential';
      | 
      | sys = bdroot; %handle for the current model ("system")
      | first = get_param(sys,'Created');
      | first = first(end-3:end);  %year is last four digits
      | 
      | last = get_param(sys,'LastModifiedDate');
      | if isempty(last)
      |     last = datestr(now,'yyyy');
      | else
      |     last = last(end-3:end);
      | end
      | 
      | if strcmp(first,last)
      |     fprintf('%s -- Copyright %s Nexteer',NxtrConf,first)
      | else
      |     fprintf('%s -- %s%s- %s Nexteer',NxtrConf,char(169),first,last)
      | end
  One : Constant  OutDataTypeStr=single
  Product2 : Product
  Reciprocal of 2 - (1/2) : Constant  Value=0.5  OutDataTypeStr=single
  Subtract : Sum  Inputs=-+
  Cos1 : Outport
  wires:
  One/1 -> Subtract/2
  Reciprocal of 2 - (1/2)/1 -> Product2/2
  Range Limited Theta Sqrd/1 -> Product2/1
  Product2/1 -> Subtract/1
  Subtract/1 -> Cos1/1

== system CM640A_MotAg1Meas/MotAg1Meas/MotAg1MeasInit1/Compute Correction Table/NVM Ok/Calculate Correction Table/Build Wave/Reconstructed Waveform Processing/Harmonic Coefficient Processing/SinCos (Use library function from NxtrMath)/Calc Range Limited Sine - 2 Term ==
  note: Sin(x) = X * (1 - X^2 * (1/6))
  note: X
  note: 1 - X^2 * (1/6)
  note: X^2 * (1/6)
  note: 1/6
  note: X^2
  note: This block calculates the taylor series of sin to 2 terms
      |
      | Sin(x) = X - X^3/3!
      | Sin(x) = X - X^3/6
      | Sin(x) = X * (1 - X^2 * (1/6))
  Range Limited Theta : Inport
  Range Limited Theta Sqrd : Inport  Port=2
  CopyRight2 : Subsystem  Description=|  mask(Copyright Information){none=on}
      | Copyright info block.                                               
      |                                                                     
      | Place copyright information at the top of every subsystem in design.
      mask prompts: none "No parameters"
      mask help: Place copyright information at the top of every subsystem in design.
      mask Display:
      | NxtrConf = 'Nexteer Confidential';
      | 
      | sys = bdroot; %handle for the current model ("system")
      | first = get_param(sys,'Created');
      | first = first(end-3:end);  %year is last four digits
      | 
      | last = get_param(sys,'LastModifiedDate');
      | if isempty(last)
      |     last = datestr(now,'yyyy');
      | else
      |     last = last(end-3:end);
      | end
      | 
      | if strcmp(first,last)
      |     fprintf('%s -- Copyright %s Nexteer',NxtrConf,first)
      | else
      |     fprintf('%s -- %s%s- %s Nexteer',NxtrConf,char(169),first,last)
      | end
  One : Constant  OutDataTypeStr=single
  Product2 : Product
  Product4 : Product
  Reciprocal of 6 - (1/6) : Constant  Value=0.166666671633720398  OutDataTypeStr=single
  Subtract : Sum  Inputs=-+
  Sin1 : Outport
  wires:
  Product4/1 -> Sin1/1
  Subtract/1 -> Product4/2
  Product2/1 -> Subtract/1
  Range Limited Theta/1 -> Product4/1
  Range Limited Theta Sqrd/1 -> Product2/1
  Reciprocal of 6 - (1/6)/1 -> Product2/2
  One/1 -> Subtract/2

== system CM640A_MotAg1Meas/MotAg1Meas/MotAg1MeasInit1/Compute Correction Table/NVM Ok/Calculate Correction Table/Build Wave/Reconstructed Waveform Processing/Harmonic Coefficient Processing/SinCos (Use library function from NxtrMath)/CopyRight2 ==

== system CM640A_MotAg1Meas/MotAg1Meas/MotAg1MeasInit1/Compute Correction Table/NVM Ok/Calculate Correction Table/Change Correction Coordinate/Waveform Coordinate Change/Correction Term Not Found/Denominator != 0/CopyRight2 ==

== system CM640A_MotAg1Meas/MotAg1Meas/MotAg1MeasInit1/Compute Correction Table/NVM Ok/Calculate Correction Table/Change Correction Coordinate/Waveform Coordinate Change/Correction Term Not Found/Denominator == 0/CopyRight2 ==
